simulink model "Q2_Van_der_Pol"  (R2026a)
settings: Solver=ode45  StopTime=30  RelTol=1e-8  AbsTol=1e-10
settings Model: Creator=szj  LastModifiedBy=szj

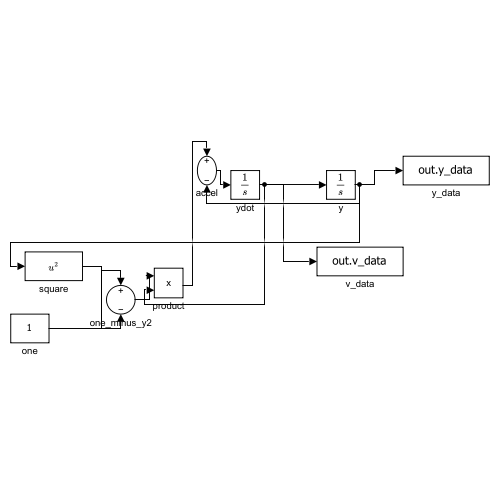
[thumbnail: Simulink's stored preview of the top-level diagram]
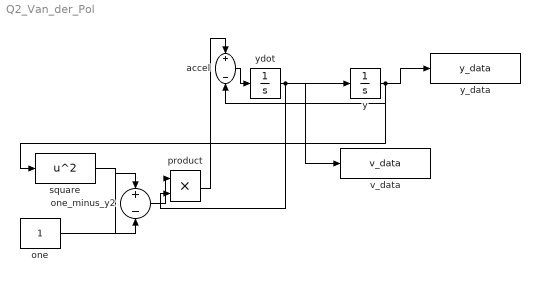
== system Q2_Van_der_Pol ==
  accel : Sum  Inputs=+-
  one : Constant
  one_minus_y2 : Sum  Inputs=+-
  product : Product
  square : Math  Operator=square
  v_data : ToWorkspace  VariableName=v_data  SaveFormat=Timeseries  SampleTime=-1
  y : Integrator  InitialCondition=2
  y_data : ToWorkspace  VariableName=y_data  SaveFormat=Timeseries  SampleTime=-1
  ydot : Integrator
  wires:
  one/1 -> one_minus_y2/1
  y/1 -> square/1, accel/2, y_data/1
  square/1 -> one_minus_y2/2
  one_minus_y2/1 -> product/1
  ydot/1 -> product/2, y/1, v_data/1
  product/1 -> accel/1
  accel/1 -> ydot/1
